simulink model "STLA_8_31"  (R2020b)
settings: Solver=ode3  StartTime=0.0  StopTime=2474  FixedStep=0.01  RelTol=1e-3
model workspace (MAT data in the model file):
  qw = 0.5
undefined symbols (not defined in the file): BSFC, continuous_torque_M, eff_speeds, eff_torques, h, km, m, m_eff, Padd, peak_torque_M, pedal_Brake, pedal_Comfort, pedal_ECO, pedal_Sport, rpm_E, rpm_M, s, speed_bp, speed_Brake, speed_Comfort, speed_ECO, speed_Sport, Tmax_eng, Topt_eng, torque_bp, torque_Brake, Torque_BSFC, torque_Comfort, torque_ECO, torque_Sport
libraries: simulink x12, svdutilitieslib x2, instrumentlib x2, autolibshared x1, aerolibconvert2 x1, pid_lib x1
(part 2 of 2)

== stateflow chart STLA_8_31/控制器/功率分配/Subsystem3/Chart ==
  state model1
    entry:
    Model=1;
  state model2
    entry:
    Model=2;
  state model3
    entry:
    Model=3;
  (default) -> model1
  model1 -> (junction 4) : [(Treq<Tm_r&SOC<0.9)==0]
  (junction 4) -> model1 [order 1] : [Treq<Tm_r&SOC<0.9]
  (junction 4) -> model2 [order 2] : [Treq>=Tm_r&SOC<0.9]
  model2 -> (junction 4) : [(Treq>=Tm_r&SOC<0.9)==0]
  (junction 4) -> model3 [order 3] : [SOC>=0.9]
  model3 -> (junction 4) : [(SOC>=0.9)==0]
  data: Treq input; Model output; Tm_r input; SOC input

== stateflow chart STLA_8_31/控制器/模式选择/Chart ==
  state Brake1
    entry:
    Model=2;
  state EV_ECO
    entry:
    Model=3;
  state stop
    entry:
    Model=1;
  state EV_Comfort
    entry:
    Model=4;
  state HEV_Sport
    entry:
    Model=8;
  state EV_Sport
    entry:
    Model=5;
  state HEV_Comfort
    entry:
    Model=7;
  state HEV_ECO
    entry:
    Model=6;
  (junction 3) -> Brake1 [order 3] : [brake>1e-4]
  Brake1 -> (junction 3) : [(brake>1e-4)==0]
  EV_ECO -> (junction 3) : [(throttle>1e-4&brake<1e-4&E_model==0&D_model==0)==0]
  (junction 3) -> EV_ECO [order 4] : [throttle>1e-4&brake<1e-4&E_model==0&D_model==0]
  (default) -> stop
  stop -> (junction 3) : [throttle>1e-4|brake>1e-4]
  (junction 3) -> stop [order 2] : [throttle<1e-4&brake<1e-4]
  (junction 3) -> HEV_Sport [order 1] : [throttle>1e-4&brake<1e-4&E_model==1&D_model==2]
  (junction 3) -> EV_Comfort [order 5] : [throttle>1e-4&brake<1e-4&E_model==0&D_model==1]
  EV_Sport -> (junction 3) : [(throttle>1e-4&brake<1e-4&E_model==0&D_model==2)==0]
  EV_Comfort -> (junction 3) : [(throttle>1e-4&brake<1e-4&E_model==0&D_model==1)==0]
  (junction 3) -> EV_Sport [order 6] : [throttle>1e-4&brake<1e-4&E_model==0&D_model==2]
  HEV_Sport -> (junction 3) : [(throttle>1e-4&brake<1e-4&E_model==1&D_model==2)==0]
  (junction 3) -> HEV_Comfort [order 8] : [throttle>1e-4&brake<1e-4&E_model==1&D_model==1]
  HEV_Comfort -> (junction 3) : [(throttle>1e-4&brake<1e-4&E_model==1&D_model==1)==0]
  HEV_ECO -> (junction 3) : [(throttle>1e-4&brake<1e-4&E_model==1&D_model==0)==0]
  (junction 3) -> HEV_ECO [order 7] : [throttle>1e-4&brake<1e-4&E_model==1&D_model==0]
  data: throttle input; brake input; Model output; E_model input; D_model input
